simulink library "GenericTarget"  (R2025b)
settings: Solver=VariableStepAuto  StartTime=0.0  StopTime=10.0  RelTol=1e-3
undefined symbols (not defined in the file or in its folder): GT_CheckUniqueParameterValue, strlength
libraries: simulink x4, $bdroot x2, etargetslib x1
(part 1 of 3)
settings Model: Creator=damerius  LastModifiedBy=damerius
settings SolverCC: AlgebraicLoopSolver=TrustRegion
settings OptimizationCC: ReuseModelBlockBuffer=off
settings DebuggingCC: UnconnectedInputMsg=warning  UnconnectedOutputMsg=warning  UnconnectedLineMsg=warning
settings ModelReferenceCC: EnableRefExpFcnMdlSchedulingChecks=on
settings RTWCC: GPUComputeCapability=3.5  DLArmComputeVersion=19.05

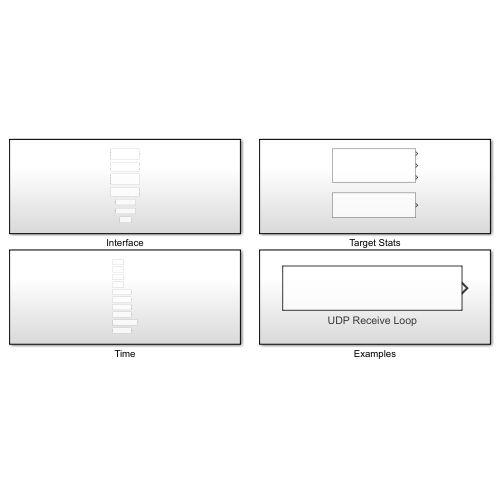
[thumbnail: Simulink's stored preview of the top-level diagram]
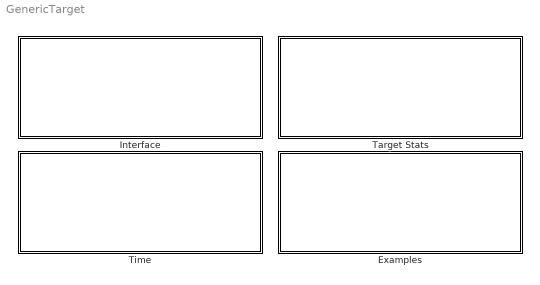
== system GenericTarget ==
  Examples : Subsystem
  Interface : Subsystem
  Target Stats : Subsystem
  Time : Subsystem

== system GenericTarget/Examples ==
  UDP Receive Loop : Subsystem  TreatAsAtomicUnit=on

== system GenericTarget/Interface ==
  Stop Execution : Subsystem  mask{SampleTime=-1}
      mask prompts: SampleTime "Sample time (-1 for inherited):"
      mask help:
      | Stop the execution of the target model. During simulation this block has no effect.<br><br>
      |
      | <b>stop</b><br>
      | True if the execution is to be stopped, false otherwise.
      mask Help: eval('GT.OpenDocumentation(''library_gt_interface_stopexecution.html'');');
      mask DialogControl DescGroupVar Prompt: Stop Execution - Generic Target
      mask Display:
      | % Get dimension of block
      | pos = get_param(gcb, 'Position');
      | width = pos(3) - pos(1);
      | height = pos(4) - pos(2);
      | 
      | % Set image to center of block
      | imgSize = 32;
      | image('GT_Icon.svg', [0.5*(width-imgSize),0.5*(height-imgSize),imgSize,imgSize]);
      | 
      | % Block title
      | text(0.5*width,0.5*(height+imgSize)+2, '{\bfStop Execution}','horizontalAlignment','center','verticalAlignment','bottom','texmode','on');
  TCP Client Receive : Subsystem  mask{showDetails=off, manageConnection=on, localPort=0, deviceName='', rxBufferSize=2048, socketPriority=6, SampleTime=-1}
      mask prompts: showDetails "Show details output port"; manageConnection "Manage connection to server"; localPort "Local port (<= 0 for dynamic port):"; deviceName "Bind to device ('' for default device):"; rxBufferSize "Receive buffer size:"; socketPriority "Socket priority (0 (lowest) ... 6 (highest), default is 6):"; SampleTime "Sample time (-1 for inherited):"
      mask help:
      | Receive data from a connected TCP server. The server address is set via the server input of a TCP Client Send or TCP Client Receive block if the <b>manageConnection</b> checkbox is enabled. For each local TCP port, a separate thread is started, that manages socket creation and connection handling to the server.<br><br>
      |
      | <b>serverAddress</b><br>A 4-dimensional vector indicating the IPv4 address of the server. A zero-value address, e.g. 0.0.0.0, disconnects the client from the server.<br><br>
      |
      | <b>serverPort</b><br>The server port. A value of 0 disconnects the client from the server.<br><br>
      |
      | <b>bytes</b><br>N-dimensional vector containing the data that has been fetched from the network buffer, where N indicates the receive buffer size.<br><br>
      |
      | <b>length</b><br>The actual number of bytes that have been received or zero in case of errors.<br><br>
      |
      | <b>details.result</b><br>Result of the socket recv function call: The number of bytes that have been received, zero if connection has been closed or a negative value in case of errors.<br><br>
      |
      | <b>details.lastErrorCode</b><br>The last socket error code from sending a message. 0 means no error. The actual meaning of non-zero values depend on the operating system.<br><br>
      |
      | <b>details.isConnected</b><br>The latest connection state to the server.
      mask init:
      | % optional details output port
      |     outPortDetails = find_system(gcb, 'LookUnderMasks','on','FollowLinks','on','Name','details');
      |     termPortDetails = find_system(gcb, 'LookUnderMasks','on','FollowLinks','on','Name','Terminator');
      |     hOut = get_param([gcb,'/BusCreator'],'PortHandles');
      |     if(showDetails)
      |         if(~isempty(termPortDetails))
      |             hIn = get_param([gcb,'/Terminator'],'PortHandles');
      |             delete_line(gcb,hOut.Outport(1),hIn.Inport(1));
      |             delete_block(termPortDetails);
      |         end
      |         if(isempty(outPortDetails))
      |             add_block('built-in/Outport',[gcb,'/details']);
      |             hIn = get_param([gcb,'/details'],'PortHandles');
      |             add_line(gcb,hOut.Outport(1),hIn.Inport(1));
      |             set_param([gcb,'/details'],'Port','3');
      |             set_param([gcb,'/details'],'Position',[25 33 55 47]);
      |         end
      |     else
      |         if(~isempty(outPortDetails))
      |             hIn = get_param([gcb,'/details'],'PortHandles');
      |             delete_line(gcb,hOut.Outport(1),hIn.Inport(1));
      |             delete_block(outPortDetails);
      |         end
      |         if(isempty(termPortDetails))
      |             add_block('built-in/Terminator',[gcb,'/Terminator']);
      |             hIn = get_param([gcb,'/Terminator'],'PortHandles');
      |             add_line(gcb,hOut.Outport(1),hIn.Inport(1));
      |             set_param([gcb,'/Terminator'],'Position',[30 30 50 50]);
      |         end
      |     end
      mask Help: eval('GT.OpenDocumentation(''library_gt_interface_tcpclientreceive.html'');');
      mask DialogControl DescGroupVar Prompt: TCP Client Receive - Generic Target
      mask DialogControl Container3 Prompt: Optional output
      mask DialogControl Container2 Prompt: Connection Management
      mask DialogControl Control2 Prompt: <i>If this checkbox is disabled, then the serverAddress and serverPort inputs are ignored.</i>
      mask DialogControl Container5 Prompt: Socket
      mask DialogControl Container6 Prompt: Advanced
      mask Display:
      | % Get dimension of block
      | pos = get_param(gcb, 'Position');
      | width = pos(3) - pos(1);
      | height = pos(4) - pos(2);
      | 
      | % Set image to center of block
      | imgSize = 32;
      | image('GT_Icon.svg', [0.5*(width-imgSize),0.5*(height-imgSize),imgSize,imgSize]);
      | 
      | % Block title
      | text(0.5*width,0.5*(height+imgSize)+2, '{\bfTCP Client Receive}','horizontalAlignment','center','verticalAlignment','bottom','texmode','on');
      | 
      | % Show socket port
      | maskStr = get_param(gcb,'localPort');
      | strText = ['Port: ' maskStr];
      | text(0.5*width,0.5*(height-imgSize)-2,strText, 'horizontalAlignment','center','verticalAlignment','top');
  TCP Client Send : Subsystem  mask{showDetails=off, manageConnection=on, localPort=0, deviceName='', socketPriority=6, SampleTime=-1}
      mask prompts: showDetails "Show details output port"; manageConnection "Manage connection to server"; localPort "Local port (<= 0 for dynamic port):"; deviceName "Bind to device ('' for default device):"; socketPriority "Socket priority (0 (lowest) ... 6 (highest), default is 6):"; SampleTime "Sample time (-1 for inherited):"
      mask help:
      | Send data to a connected TCP server. The server address is set via the server input of a TCP Client Send or TCP Client Receive block if the <b>manageConnection</b> checkbox is enabled. For each local TCP port, a separate thread is started, that manages socket creation and connection handling to the server.<br><br>
      |
      | <b>serverAddress</b><br>A 4-dimensional vector indicating the IPv4 address of the server. A zero-value address, e.g. 0.0.0.0, disconnects the client from the server.<br><br>
      |
      | <b>serverPort</b><br>The server port. A value of 0 disconnects the client from the server.<br><br>
      |
      | <b>bytes</b><br>A vector containing the data that should be sent.<br><br>
      |
      | <b>length</b><br>The number of bytes that should be sent.<br><br>
      |
      | <b>numBytesSent</b><br>The number of bytes that have been sent or zero in case of errors.<br><br>
      |
      | <b>details.result</b><br>Result of the socket send function call: The number of bytes that have been sent or a negative value in case of errors.<br><br>
      |
      | <b>details.lastErrorCode</b><br>The last socket error code from sending a message. 0 means no error. The actual meaning of non-zero values depend on the operating system.<br><br>
      |
      | <b>details.isConnected</b><br>The latest connection state to the server.
      mask init:
      | outPortDetails = find_system(gcb, 'LookUnderMasks','on','FollowLinks','on','Name','details');
      |     termPortDetails = find_system(gcb, 'LookUnderMasks','on','FollowLinks','on','Name','Terminator');
      |     hOut = get_param([gcb,'/BusCreator'],'PortHandles');
      |     if(showDetails)
      |         if(~isempty(termPortDetails))
      |             hIn = get_param([gcb,'/Terminator'],'PortHandles');
      |             delete_line(gcb,hOut.Outport(1),hIn.Inport(1));
      |             delete_block(termPortDetails);
      |         end
      |         if(isempty(outPortDetails))
      |             add_block('built-in/Outport',[gcb,'/details']);
      |             hIn = get_param([gcb,'/details'],'PortHandles');
      |             add_line(gcb,hOut.Outport(1),hIn.Inport(1));
      |             set_param([gcb,'/details'],'Port','2');
      |             set_param([gcb,'/details'],'Position',[10 33 40 47]);
      |         end
      |     else
      |         if(~isempty(outPortDetails))
      |             hIn = get_param([gcb,'/details'],'PortHandles');
      |             delete_line(gcb,hOut.Outport(1),hIn.Inport(1));
      |             delete_block(outPortDetails);
      |         end
      |         if(isempty(termPortDetails))
      |             add_block('built-in/Terminator',[gcb,'/Terminator']);
      |             hIn = get_param([gcb,'/Terminator'],'PortHandles');
      |             add_line(gcb,hOut.Outport(1),hIn.Inport(1));
      |             set_param([gcb,'/Terminator'],'Position',[15 30 35 50]);
      |         end
      |     end
      mask Help: eval('GT.OpenDocumentation(''library_gt_interface_tcpclientsend.html'');');
      mask DialogControl DescGroupVar Prompt: TCP Client Send - Generic Target
      mask DialogControl Container7 Prompt: Optional output
      mask DialogControl Container6 Prompt: Connection Management
      mask DialogControl Control2 Prompt: <i>If this checkbox is disabled, then the serverAddress and serverPort inputs are ignored.</i>
      mask DialogControl Container4 Prompt: Socket
      mask DialogControl Container5 Prompt: Advanced
      mask Display:
      | % Get dimension of block
      | pos = get_param(gcb, 'Position');
      | width = pos(3) - pos(1);
      | height = pos(4) - pos(2);
      | 
      | % Set image to center of block
      | imgSize = 32;
      | image('GT_Icon.svg', [0.5*(width-imgSize),0.5*(height-imgSize),imgSize,imgSize]);
      | 
      | % Block title
      | text(0.5*width,0.5*(height+imgSize)+2, '{\bfTCP Client Send}','horizontalAlignment','center','verticalAlignment','bottom','texmode','on');
      | 
      | % Show socket port
      | maskStr = get_param(gcb,'localPort');
      | strText = ['Port: ' maskStr];
      | text(0.5*width,0.5*(height-imgSize)-2,strText, 'horizontalAlignment','center','verticalAlignment','top');
  UDP Receive : Subsystem  mask{showDetails=off, localPort=0, deviceName='', rxBufferSize=2048, multicastGroupSource=internal, multicastGroup=[0,0,0,0], multicastTTL=1, multicastInterfaceAddress=[0,0,0,0], multicastAll=on, multicastLoop=on, socketPriority=6, allowBroadcast=off, allowZeroLengthMessage=off, fetchAll=on, SampleTime=-1}
      mask prompts: showDetails "Show details output port"; localPort "Local port (<= 0 for dynamic port):"; deviceName "Bind to device ('' for default device):"; rxBufferSize "Receive buffer size:"; multicastGroupSource "Multicast group source:"; multicastGroup "Multicast groups to join (N-by-4 matrix):"; multicastTTL "Time-to-live value for outgoing multicast traffic (default is 1):"; multicastInterfaceAddress "Multicast interface address ([0,0,0,0] for INADDR_ANY):"; multicastAll "IP_MULTICAST_ALL"; multicastLoop "IP_MULTICAST_LOOP"; socketPriority "Socket priority (0 (lowest) ... 6 (highest), default is 6):"; allowBroadcast "Allow sending broadcast message"; allowZeroLengthMessage "Allow sending zero-length message"; fetchAll "Fetch all messages from the network buffer"; SampleTime "Sample time (-1 for inherited):"
      mask help:
      | Receive a UDP message at the specified port. By default all messages from the network buffer of the operating system are fetched and only the latest message is returned. However, this option can be disabled in the advanced tab.<br><br>
      |
      | <b>bytes</b><br>N-dimensional vector containing the latest message that has been fetched from the network buffer, where N indicates the receive buffer size.<br><br>
      |
      | <b>length</b><br>The actual length of the corresponding message or zero in case of errors.<br><br>
      |
      | <b>details.sourceAddress</b><br>A 4-dimensional vector denoting the IPv4 source address of the received message.<br><br>
      |
      | <b>details.sourcePort</b><br>The source port of the received message.<br><br>
      |
      | <b>details.result</b><br>Result of the socket recvfrom function call: The number of bytes that have been received or a negative value in case of errors.<br><br>
      |
      | <b>details.lastErrorCode</b><br>The last socket error code from receiving a message. 0 means no error. The actual meaning of non-zero values depend on the operating system.<br><br>
      |
      | <b>groupsToJoin</b><br>Optional input that is enabled if the multicast group source is set to external in the multicast tab. The signal must be an N-by-4 matrix that represent N multicast group addresses to be joined. Addresses not being inside the valid multicast group address range are ignored.
      mask init:
      | % optional details output port
      |     outPortDetails = find_system(gcb, 'LookUnderMasks','on','FollowLinks','on','Name','details');
      |     termPortDetails = find_system(gcb, 'LookUnderMasks','on','FollowLinks','on','Name','Terminator');
      |     hOut = get_param([gcb,'/BusCreator'],'PortHandles');
      |     if(showDetails)
      |         if(~isempty(termPortDetails))
      |             hIn = get_param([gcb,'/Terminator'],'PortHandles');
      |             delete_line(gcb,hOut.Outport(1),hIn.Inport(1));
      |             delete_block(termPortDetails);
      |         end
      |         if(isempty(outPortDetails))
      |             add_block('built-in/Outport',[gcb,'/details']);
      |             hIn = get_param([gcb,'/details'],'PortHandles');
      |             add_line(gcb,hOut.Outport(1),hIn.Inport(1));
      |             set_param([gcb,'/details'],'Port','3');
      |             set_param([gcb,'/details'],'Position',[25 33 55 47]);
      |         end
      |     else
      |         if(~isempty(outPortDetails))
      |             hIn = get_param([gcb,'/details'],'PortHandles');
      |             delete_line(gcb,hOut.Outport(1),hIn.Inport(1));
      |             delete_block(outPortDetails);
      |         end
      |         if(isempty(termPortDetails))
      |             add_block('built-in/Terminator',[gcb,'/Terminator']);
      |             hIn = get_param([gcb,'/Terminator'],'PortHandles');
      |             add_line(gcb,hOut.Outport(1),hIn.Inport(1));
      |             set_param([gcb,'/Terminator'],'Position',[30 30 50 50]);
      |         end
      |     end
      | 
      |     % multicastGroups input port
      |     inPortGroups = find_system(gcb, 'LookUnderMasks','on','FollowLinks','on','Name','groupsToJoin');
      |     constantGroups = find_system(gcb, 'LookUnderMasks','on','FollowLinks','on','Name','constantGroupsToJoin');
      |     popupValue = get_param(gcb,'multicastGroupSource');
      |     hIn = get_param([gcb,'/Transpose'],'PortHandles');
      |     if(strcmp(popupValue,'internal'))
      |         if(~isempty(inPortGroups))
      |             hOut = get_param([gcb,'/groupsToJoin'],'PortHandles');
      |             delete_line(gcb,hOut.Outport(1),hIn.Inport(1));
      |             delete_block(inPortGroups);
      |         end
      |         if(isempty(constantGroups))
      |             add_block('built-in/Constant',[gcb,'/constantGroupsToJoin']);
      |             hOut = get_param([gcb,'/constantGroupsToJoin'],'PortHandles');
      |             add_line(gcb,hOut.Outport(1),hIn.Inport(1));
      |             set_param([gcb,'/constantGroupsToJoin'],'Value','multicastGroup');
      |             set_param([gcb,'/constantGroupsToJoin'],'Position',[-1290 -5 -1120 15]);
      |         end
      |     else
      |         if(~isempty(constantGroups))
      |             hOut = get_param([gcb,'/constantGroupsToJoin'],'PortHandles');
      |             delete_line(gcb,hOut.Outport(1),hIn.Inport(1));
      |             delete_block(constantGroups);
      |         end
      |         if(isempty(inPortGroups))
      |             add_block('built-in/Inport',[gcb,'/groupsToJoin']);
      |             hOut = get_param([gcb,'/groupsToJoin'],'PortHandles');
      |             add_line(gcb,hOut.Outport(1),hIn.Inport(1));
      |             set_param([gcb,'/groupsToJoin'],'Port','1');
      |             set_param([gcb,'/groupsToJoin'],'Position',[-1150 -2 -1120 12]);
      |         end
      |     end
      mask Help: eval('GT.OpenDocumentation(''library_gt_interface_udpreceive.html'');');
      mask Callback multicastGroupSource:
      | popupValue = get_param(gcb,'multicastGroupSource');
      |     if(strcmp(popupValue, 'internal'))
      |         set_param(gcb,'MaskEnables',{'on','on','on','on','on','on','on','on','on','on','on','on','on','on','on'});
      |     else
      |         set_param(gcb,'MaskEnables',{'on','on','on','on','on','off','on','on','on','on','on','on','on','on','on'});
      |     end
      mask DialogControl DescGroupVar Prompt: UDP Receive - Generic Target
      mask DialogControl ParameterGroupVar Prompt: Optional output
      mask DialogControl Container4 Prompt: Socket
      mask DialogControl Container5 Prompt: Multicast
      mask DialogControl Container7 Prompt: Socket options
      mask DialogControl Container6 Prompt: Advanced
      mask Display:
      | % Get dimension of block
      | pos = get_param(gcb, 'Position');
      | width = pos(3) - pos(1);
      | height = pos(4) - pos(2);
      | 
      | % Set image to center of block
      | imgSize = 32;
      | image('GT_Icon.svg', [0.5*(width-imgSize),0.5*(height-imgSize),imgSize,imgSize]);
      | 
      | % Block title
      | text(0.5*width,0.5*(height+imgSize)+2, '{\bfUDP Receive}','horizontalAlignment','center','verticalAlignment','bottom','texmode','on');
      | 
      | % Show socket port
      | maskStr = get_param(gcb,'localPort');
      | strText = ['Port: ' maskStr];
      | text(0.5*width,0.5*(height-imgSize)-2,strText, 'horizontalAlignment','center','verticalAlignment','top');
  UDP Send : Subsystem  mask{showDetails=off, localPort=0, deviceName='', multicastTTL=1, multicastInterfaceAddress=[0,0,0,0], multicastAll=on, multicastLoop=on, socketPriority=6, allowBroadcast=off, allowZeroLengthMessage=off, SampleTime=-1}
      mask prompts: showDetails "Show details output port"; localPort "Local port (<= 0 for dynamic port):"; deviceName "Bind to device ('' for default device):"; multicastTTL "Time-to-live value for outgoing multicast traffic (default is 1):"; multicastInterfaceAddress "Multicast interface address ([0,0,0,0] for INADDR_ANY):"; multicastAll "IP_MULTICAST_ALL"; multicastLoop "IP_MULTICAST_LOOP"; socketPriority "Socket priority (0 (lowest) ... 6 (highest), default is 6):"; allowBroadcast "Allow sending broadcast message"; allowZeroLengthMessage "Allow sending zero-length message"; SampleTime "Sample time (-1 for inherited):"
      mask help:
      | Send a UDP message to a destination address that is specified via the destination input. By default a message of zero-length is not sent. However, this option can be enabled in the advanced tab.<br><br>
      |
      | <b>destinationAddress</b><br>A 4-dimensional vector indicating the destination IPv4 address.<br><br>
      |
      | <b>destinationPort</b><br>The destination port.<br><br>
      |
      | <b>bytes</b><br>A vector containing the message that should be sent.<br><br>
      |
      | <b>length</b><br>The number of bytes that should be sent. The length must not be greater than 65507.<br><br>
      |
      | <b>details.result</b><br>Result of the socket sendto function call: The number of bytes that have been sent or a negative value in case of errors.<br><br>
      |
      | <b>details.lastErrorCode</b><br>The last socket error code from sending a message. 0 means no error. The actual meaning of non-zero values depend on the operating system.
      mask init:
      | outPortDetails = find_system(gcb, 'LookUnderMasks','on','FollowLinks','on','Name','details');
      |     termPortDetails = find_system(gcb, 'LookUnderMasks','on','FollowLinks','on','Name','Terminator');
      |     hOut = get_param([gcb,'/BusCreator'],'PortHandles');
      |     if(showDetails)
      |         if(~isempty(termPortDetails))
      |             hIn = get_param([gcb,'/Terminator'],'PortHandles');
      |             delete_line(gcb,hOut.Outport(1),hIn.Inport(1));
      |             delete_block(termPortDetails);
      |         end
      |         if(isempty(outPortDetails))
      |             add_block('built-in/Outport',[gcb,'/details']);
      |             hIn = get_param([gcb,'/details'],'PortHandles');
      |             add_line(gcb,hOut.Outport(1),hIn.Inport(1));
      |             set_param([gcb,'/details'],'Port','1');
      |             set_param([gcb,'/details'],'Position',[10 33 40 47]);
      |         end
      |     else
      |         if(~isempty(outPortDetails))
      |             hIn = get_param([gcb,'/details'],'PortHandles');
      |             delete_line(gcb,hOut.Outport(1),hIn.Inport(1));
      |             delete_block(outPortDetails);
      |         end
      |         if(isempty(termPortDetails))
      |             add_block('built-in/Terminator',[gcb,'/Terminator']);
      |             hIn = get_param([gcb,'/Terminator'],'PortHandles');
      |             add_line(gcb,hOut.Outport(1),hIn.Inport(1));
      |             set_param([gcb,'/Terminator'],'Position',[15 30 35 50]);
      |         end
      |     end
      mask Help: eval('GT.OpenDocumentation(''library_gt_interface_udpsend.html'');');
      mask DialogControl DescGroupVar Prompt: UDP Send - Generic Target
      mask DialogControl ParameterGroupVar Prompt: Optional output
      mask DialogControl Container4 Prompt: Socket
      mask DialogControl Container6 Prompt: Multicast
      mask DialogControl Container7 Prompt: Socket options
      mask DialogControl Container5 Prompt: Advanced
      mask Display:
      | % Get dimension of block
      | pos = get_param(gcb, 'Position');
      | width = pos(3) - pos(1);
      | height = pos(4) - pos(2);
      | 
      | % Set image to center of block
      | imgSize = 32;
      | image('GT_Icon.svg', [0.5*(width-imgSize),0.5*(height-imgSize),imgSize,imgSize]);
      | 
      | % Block title
      | text(0.5*width,0.5*(height+imgSize)+2, '{\bfUDP Send}','horizontalAlignment','center','verticalAlignment','bottom','texmode','on');
      | 
      | % Show socket port
      | maskStr = get_param(gcb,'localPort');
      | strText = ['Port: ' maskStr];
      | text(0.5*width,0.5*(height-imgSize)-2,strText, 'horizontalAlignment','center','verticalAlignment','top');
  Write Bus To File : Subsystem  InitFcn=GT_CheckUniqueParameterValue(gcs,gcb,'strID');  mask{strID='myData', numSamplesPerFile=0, threadPriority=30, writeFilesDuringSimulation=off, SampleTime=-1, numBytesPerSample=8, strSignalNames='a', strlenSignalNames=1, strDimensions='[1]', strlenDimensions=3, strDataTypes='double', strlenDataTypes=6}
      mask prompts: strID "Unique ID:"; numSamplesPerFile "Number of samples per file (0 for infinite samples):"; threadPriority "Thread priority in range [1 (lowest), 99 (highest)]:"; writeFilesDuringSimulation "write files during simulation"; SampleTime "Sample time (-1 for inherited):"
      mask help: Write a complete bus signal to a file. Internally a digital clock is used as timestamp. The number of samples to be written into a single file can be specified. A sample indicates a data vector of all signals in the bus and the timestamp for one sample time point.
      mask init:
      | GT_WriteBusToFileInitFcn(gcb);
      mask Help: eval('GT.OpenDocumentation(''library_gt_interface_writebustofile.html'');');
      mask DialogControl DescGroupVar Prompt: Write Bus To File - Generic Target
      mask DialogControl Container3 Prompt: Bus input
      mask DialogControl Control3 Prompt: Connect a bus signal to the input port and click the "Update" button. Make sure that the model can be compiled successfully.
      mask DialogControl buttonUpdate Prompt: Update
      mask DialogControl buttonUpdate Callback: GT_UpdateWriteBusToFile(gcb);
      mask DialogControl Control4 Prompt: <p style="color: #f00;"><b>NOTE:</b> You must not use multiple Write To File blocks with the <u>same</u> ID!</p>
      mask DialogControl Control5 Prompt: If this option is enabled, a data folder is created to the current working directory whenever the initialization callback is triggered.
      mask DialogControl Container5 Prompt: Hidden Parameters
      mask Display:
      | % Get dimension of block
      | pos = get_param(gcb, 'Position');
      | width = pos(3) - pos(1);
      | height = pos(4) - pos(2);
      | 
      | % Set image to center of block
      | imgSize = 32;
      | image('GT_Icon.svg', [0.5*(width-imgSize),0.5*(height-imgSize),imgSize,imgSize]);
      | 
      | % Block title
      | text(0.5*width,0.5*(height+imgSize)+2, '{\bfWrite Bus To File}','horizontalAlignment','center','verticalAlignment','bottom','texmode','on');
      | 
      | % Show ID
      | maskStr = get_param(gcb,'strID');
      | text(4,2,['ID: ',maskStr],'horizontalAlignment','left','verticalAlignment','bottom');
  Write Scalar Doubles To File : Subsystem  InitFcn=GT_CheckUniqueParameterValue(gcs,gcb,'strID');  mask{strID='myData', numSamplesPerFile=0, threadPriority=30, writeFilesDuringSimulation=off, numSignals=2, signalNames=signal1,signal2, numCharacters=15, SampleTime=-1}
      mask prompts: strID "Unique ID:"; numSamplesPerFile "Number of samples per file (0 for infinite samples):"; threadPriority "Thread priority in range [1 (lowest), 99 (highest)]:"; writeFilesDuringSimulation "write files during simulation"; SampleTime "Sample time (-1 for inherited):"
      mask help:
      | Write a bus signal of scalar doubles to a file. Internally, a digital clock is used as timestamp. The number of samples to be written into one file can be specified. A sample indicates a vector of values including the time and all signals in the bus.<br>
      | <p style="color: #f00;"><b>NOTE:</b> The input <u>must</u> be connected to a bus that only contains scalar values of type double! Otherwise, the mask initialization function is going to fail.</p>
      | If structural changes have been made to the input bus, it may be necessary to update the model twice.
      mask init:
      | GT_WriteScalarDoublesToFileInitFcn(gcb);
      mask Help: eval('GT.OpenDocumentation(''library_gt_interface_writescalardoublestofile.html'');');
      mask DialogControl DescGroupVar Prompt: Write Scalar Doubles To File - Generic Target
      mask DialogControl Control2 Prompt: <p style="color: #f00;"><b>NOTE:</b> You must not use multiple Write To File blocks with the <u>same</u> ID!</p>
      mask DialogControl Control3 Prompt: If this option is enabled, a data folder is created to the current working directory whenever the initialization callback is triggered.
      mask Display:
      | % Get dimension of block
      | pos = get_param(gcb, 'Position');
      | width = pos(3) - pos(1);
      | height = pos(4) - pos(2);
      | 
      | % Set image to center of block
      | imgSize = 32;
      | image('GT_Icon.svg', [0.5*(width-imgSize),0.5*(height-imgSize),imgSize,imgSize]);
      | 
      | % Block title
      | text(0.5*width,0.5*(height+imgSize)+2, '{\bfWrite Scalar Doubes To File}','horizontalAlignment','center','verticalAlignment','bottom','texmode','on');
      | 
      | % Show ID
      | maskStr = get_param(gcb,'strID');
      | text(4,2,['ID: ',maskStr],'horizontalAlignment','left','verticalAlignment','bottom');

== system GenericTarget/Target Stats ==
  Application Arguments : Subsystem  mask{maxNumCharsPerArgument=32, maxNumArguments=8, SampleTime=-1}
      mask prompts: maxNumCharsPerArgument "Maximum number of characters per argument:"; maxNumArguments "Maximum number of arguments:"; SampleTime "Sample time (-1 for inherited):"
      mask help:
      | Get all arguments that have been passed to the application. The first argument is the executable name. The maximum number of characters as well as the maximum number of arguments that can be stored in the output are configured via the block mask. During simulation this block has no effect.<br><br>
      | <b>args</b><br>
      | N-by-M matrix of type uint8, where N and M indicate the maximum number of characters per argument and the maximum number of arguments, respectively.
      | <br><br>
      | <b>numCharacters</b><br>
      | M-dimensional vector of type uint32, where each element indicates the actual number of characters that represent the argument in the M-th column of the <i>args</i> output matrix.
      | <br><br>
      | <b>numArguments</b><br>
      | Scalar value of type uint32 indicating the actual number of arguments present in the <i>args</i> output matrix.
      mask Help: eval('GT.OpenDocumentation(''library_gt_targetstats_applicationarguments.html'');');
      mask DialogControl DescGroupVar Prompt: Application Arguments
      mask Display:
      | % Get dimension of block
      | pos = get_param(gcb, 'Position');
      | width = pos(3) - pos(1);
      | height = pos(4) - pos(2);
      | 
      | % Set image to center of block
      | imgSize = 32;
      | image('GT_Icon.svg', [0.5*(width-imgSize),0.5*(height-imgSize),imgSize,imgSize]);
      | 
      | % Block title
      | text(width/2, height, '{\bfApplication Arguments}','horizontalAlignment','center','verticalAlignment','top','texmode','on');
  Read Thermal Zones : Subsystem  mask{maxNumThermalZones=8, SampleTime=-1}
      mask prompts: maxNumThermalZones "Maximum number of thermal zones:"; SampleTime "Sample time (-1 for inherited):"
      mask help: Read all temperature values from "/sys/class/thermal/thermal_zone[i]/temp" with [i] being the index of the thermal zone. The maximum number of thermal zones to read from is specified via the mask parameter. The output dimension is equal to that number. If a thermal zone does not exist, NaN is returned for the corresponding index. This block has no effect on a non-linux OS.
      mask Help: eval('GT.OpenDocumentation(''library_gt_targetstats_readthermalzones.html'');');
      mask DialogControl DescGroupVar Prompt: Read Thermal Zones - Generic Target
      mask Display:
      | % Get dimension of block
      | pos = get_param(gcb, 'Position');
      | width = pos(3) - pos(1);
      | height = pos(4) - pos(2);
      | 
      | % Set image to center of block
      | imgSize = 32;
      | image('GT_Icon.svg', [0.5*(width-imgSize),0.5*(height-imgSize),imgSize,imgSize]);
      | 
      | % Block title
      | text(width/2, height, '{\bfRead Thermal Zones}','horizontalAlignment','center','verticalAlignment','top','texmode','on');

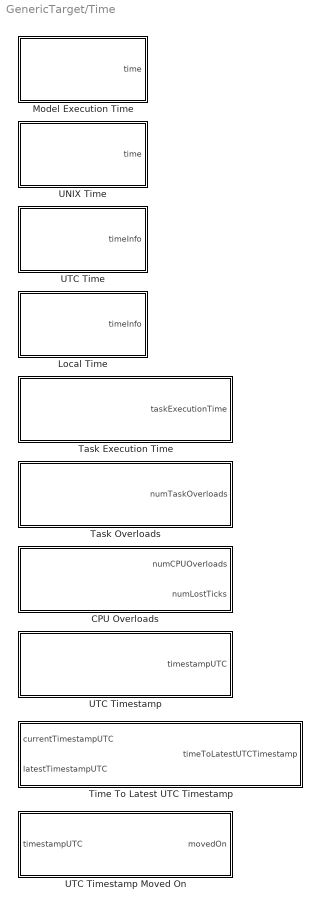
== system GenericTarget/Time ==
  CPU Overloads : Subsystem  mask{SampleTime=-1}
      mask prompts: SampleTime "Sample time (-1 for inherited):"
      mask help:
      | Get the total number of CPU overloads and lost ticks since the model has been started. During simulation this block has no effect.<br><br>
      | <b>numCPUOverloads</b><br>
      | The total number of CPU overloads that have been occurred. This value is incremented by one, if the timer interrupt event for the base rate scheduler (with the base sampletime of the model) has been lost.
      | <br><br>
      | <b>numLostTicks</b><br>
      | The total number of lost ticks from the timer. This value is incremented by the number of lost timer interrupt events.
      mask Help: eval('GT.OpenDocumentation(''library_gt_time_cpuoverloads.html'');');
      mask DialogControl DescGroupVar Prompt: CPU Overloads - Generic Target
      mask Display:
      | % Get dimension of block
      | pos = get_param(gcb, 'Position');
      | width = pos(3) - pos(1);
      | height = pos(4) - pos(2);
      | 
      | % Set image to center of block
      | imgSize = 32;
      | image('GT_Icon.svg', [0.5*(width-imgSize),0.5*(height-imgSize),imgSize,imgSize]);
      | 
      | % Block title
      | text(width/2, height, '{\bfCPU Overloads}','horizontalAlignment','center','verticalAlignment','top','texmode','on');
  Local Time : Subsystem  mask{SampleTime=-1}
      mask prompts: SampleTime "Sample time (-1 for inherited):"
      mask help:
      | Get the current local time from the system clock.<br><br>
      |
      | <b>timeInfo.nanoseconds</b><br>Nanoseconds after the second [0, 999999999].<br><br>
      |
      | <b>timeInfo.second</b><br>Seconds after the minute [0, 59] (on some systems [0,60] or [0,61] to allow leap seconds).<br><br>
      |
      | <b>timeInfo.minute</b><br>Minutes after the hour [0, 59].<br><br>
      |
      | <b>timeInfo.hour</b><br>Hours since midnight [0, 23].<br><br>
      |
      | <b>timeInfo.mday</b><br>Day of the month [1, 31].<br><br>
      |
      | <b>timeInfo.mon</b><br>Month since January [0, 11].<br><br>
      |
      | <b>timeInfo.year</b><br>Years since 1900.<br><br>
      |
      | <b>timeInfo.wday</b><br>Days since Sunday [0, 6].<br><br>
      |
      | <b>timeInfo.yday</b><br>Days since January 1 [0, 365].<br><br>
      |
      | <b>timeInfo.isdst</b><br>Daylight Saving Time flag. The value is positive if DST is in effect, zero if not and negative if no information is available.
      mask Help: eval('GT.OpenDocumentation(''library_gt_time_localtime.html'');');
      mask DialogControl DescGroupVar Prompt: Local Time - Generic Target
      mask Display:
      | % Get dimension of block
      | pos = get_param(gcb, 'Position');
      | width = pos(3) - pos(1);
      | height = pos(4) - pos(2);
      | 
      | % Set image to center of block
      | imgSize = 32;
      | image('GT_Icon.svg', [0.5*(width-imgSize),0.5*(height-imgSize),imgSize,imgSize]);
      | 
      | % Block title
      | text(width/2, height, '{\bfLocal Time}','horizontalAlignment','center','verticalAlignment','top','texmode','on');
  Model Execution Time : Subsystem  mask{SampleTime=-1}
      mask prompts: SampleTime "Sample time (-1 for inherited):"
      mask help:
      | Get the current model execution time. A steady clock is used to measure the execution time, that is, the elapsed time to the starting timepoint of the scheduler. During simulation, the output represents the measured time to some initial timepoint at the start of the simulation.<br><br>
      |
      | <b>time</b><br>The model execution time in seconds.
      mask Help: eval('GT.OpenDocumentation(''library_gt_time_modelexecutiontime.html'');');
      mask DialogControl DescGroupVar Prompt: Model Execution Time - Generic Target
      mask Display:
      | % Get dimension of block
      | pos = get_param(gcb, 'Position');
      | width = pos(3) - pos(1);
      | height = pos(4) - pos(2);
      | 
      | % Set image to center of block
      | imgSize = 32;
      | image('GT_Icon.svg', [0.5*(width-imgSize),0.5*(height-imgSize),imgSize,imgSize]);
      | 
      | % Block title
      | text(width/2, height, '{\bfModel Execution Time}','horizontalAlignment','center','verticalAlignment','top','texmode','on');
  Task Execution Time : Subsystem  mask{strTaskName='D1', SampleTime=-1}
      mask prompts: strTaskName "Task name, e.g. 'D1':"; SampleTime "Sample time (-1 for inherited):"
      mask help: Get the current task execution time in seconds for the task with the specified name. If this task does not exist, zero is returned. During simulation this block has no effect.
      mask Help: eval('GT.OpenDocumentation(''library_gt_time_taskexecutiontime.html'');');
      mask DialogControl DescGroupVar Prompt: Task Execution Time - Generic Target
      mask Display:
      | % Get dimension of block
      | pos = get_param(gcb, 'Position');
      | width = pos(3) - pos(1);
      | height = pos(4) - pos(2);
      | 
      | % Set image to center of block
      | imgSize = 32;
      | image('GT_Icon.svg', [0.5*(width-imgSize),0.5*(height-imgSize),imgSize,imgSize]);
      | 
      | % Block title
      | text(width/2, height, '{\bfTask Execution Time}','horizontalAlignment','center','verticalAlignment','top','texmode','on');
      | 
      | % Show task name
      | maskStr = get_param(gcb,'strTaskName');
      | text(4,2,['Task: ',maskStr],'horizontalAlignment','left','verticalAlignment','bottom');
  Task Overloads : Subsystem  mask{strTaskName='D1', SampleTime=-1}
      mask prompts: strTaskName "Task name, e.g. 'D1':"; SampleTime "Sample time (-1 for inherited):"
      mask help: Get the total number of task overloads for the task with the specified name. If this task does not exist, zero is returned. During simulation this block has no effect.
      mask Help: eval('GT.OpenDocumentation(''library_gt_time_taskoverloads.html'');');
      mask DialogControl DescGroupVar Prompt: Task Overloads - Generic Target
      mask Display:
      | % Get dimension of block
      | pos = get_param(gcb, 'Position');
      | width = pos(3) - pos(1);
      | height = pos(4) - pos(2);
      | 
      | % Set image to center of block
      | imgSize = 32;
      | image('GT_Icon.svg', [0.5*(width-imgSize),0.5*(height-imgSize),imgSize,imgSize]);
      | 
      | % Block title
      | text(width/2, height, '{\bfTask Overloads}','horizontalAlignment','center','verticalAlignment','top','texmode','on');
      | 
      | % Show task name
      | maskStr = get_param(gcb,'strTaskName');
      | text(4,2,['Task: ',maskStr],'horizontalAlignment','left','verticalAlignment','bottom');
  Time To Latest UTC Timestamp : Subsystem
      mask help:
      | This block calculates the time difference (seconds) to the latest UTC timestamp taking into account the wrap range of the UTC timestamp.<br><br>
      | The basic behaviour is as follows:<br>
      | <b>output</b> = <b>current</b> - <b>latest</b>
      mask Help: eval('GT.OpenDocumentation(''library_gt_time_timetolatestutctimestamp.html'');');
      mask DialogControl DescGroupVar Prompt: Time To Latest UTC Timestamp - Generic Target
      mask Display:
      | % Get dimension of block
      | pos = get_param(gcb, 'Position');
      | width = pos(3) - pos(1);
      | height = pos(4) - pos(2);
      | 
      | % Set image to center of block
      | imgSize = 32;
      | image('GT_Icon.svg', [0.5*(width-imgSize),0.5*(height-imgSize),imgSize,imgSize]);
      | 
      | % Block title
      | text(width/2, height, '{\bfTime To Latest UTC Timestamp}','horizontalAlignment','center','verticalAlignment','top','texmode','on');
  UNIX Time : Subsystem  mask{SampleTime=-1}
      mask prompts: SampleTime "Sample time (-1 for inherited):"
      mask help:
      | Get the current UNIX time from the system clock.<br><br>
      |
      | <b>time</b><br>The UNIX time in seconds. The resolution is one millisecond.
      mask Help: eval('GT.OpenDocumentation(''library_gt_time_unixtime.html'');');
      mask DialogControl DescGroupVar Prompt: UNIX Time - Generic Target
      mask Display:
      | % Get dimension of block
      | pos = get_param(gcb, 'Position');
      | width = pos(3) - pos(1);
      | height = pos(4) - pos(2);
      | 
      | % Set image to center of block
      | imgSize = 32;
      | image('GT_Icon.svg', [0.5*(width-imgSize),0.5*(height-imgSize),imgSize,imgSize]);
      | 
      | % Block title
      | text(width/2, height, '{\bfUNIX Time}','horizontalAlignment','center','verticalAlignment','top','texmode','on');
  UTC Time : Subsystem  mask{SampleTime=-1}
      mask prompts: SampleTime "Sample time (-1 for inherited):"
      mask help:
      | Get the current UTC time from the system clock.<br><br>
      |
      | <b>timeInfo.nanoseconds</b><br>Nanoseconds after the second [0, 999999999].<br><br>
      |
      | <b>timeInfo.second</b><br>Seconds after the minute [0, 59] (on some systems [0,60] or [0,61] to allow leap seconds).<br><br>
      |
      | <b>timeInfo.minute</b><br>Minutes after the hour [0, 59].<br><br>
      |
      | <b>timeInfo.hour</b><br>Hours since midnight [0, 23].<br><br>
      |
      | <b>timeInfo.mday</b><br>Day of the month [1, 31].<br><br>
      |
      | <b>timeInfo.mon</b><br>Month since January [0, 11].<br><br>
      |
      | <b>timeInfo.year</b><br>Years since 1900.<br><br>
      |
      | <b>timeInfo.wday</b><br>Days since Sunday [0, 6].<br><br>
      |
      | <b>timeInfo.yday</b><br>Days since January 1 [0, 365].<br><br>
      |
      | <b>timeInfo.isdst</b><br>Daylight Saving Time flag. The value is positive if DST is in effect, zero if not and negative if no information is available.
      mask Help: eval('GT.OpenDocumentation(''library_gt_time_utctime.html'');');
      mask DialogControl DescGroupVar Prompt: UTC Time - Generic Target
      mask Display:
      | % Get dimension of block
      | pos = get_param(gcb, 'Position');
      | width = pos(3) - pos(1);
      | height = pos(4) - pos(2);
      | 
      | % Set image to center of block
      | imgSize = 32;
      | image('GT_Icon.svg', [0.5*(width-imgSize),0.5*(height-imgSize),imgSize,imgSize]);
      | 
      | % Block title
      | text(width/2, height, '{\bfUTC Time}','horizontalAlignment','center','verticalAlignment','top','texmode','on');
  UTC Timestamp : Subsystem  mask{SampleTime=-1}
      mask prompts: SampleTime "Sample time (-1 for inherited):"
      mask help:
      | Get the current UTC timestamp from the system clock.<br><br>
      |
      | <b>timestampUTC</b><br>UTC second of the day in range [0,86400) (on some systems [0,86401) or [0,86402) to allow leap seconds).
      mask Help: eval('GT.OpenDocumentation(''library_gt_time_utctimestamp.html'');');
      mask DialogControl DescGroupVar Prompt: UTC Timestamp - Generic Target
      mask Display:
      | % Get dimension of block
      | pos = get_param(gcb, 'Position');
      | width = pos(3) - pos(1);
      | height = pos(4) - pos(2);
      | 
      | % Set image to center of block
      | imgSize = 32;
      | image('GT_Icon.svg', [0.5*(width-imgSize),0.5*(height-imgSize),imgSize,imgSize]);
      | 
      | % Block title
      | text(width/2, height, '{\bfUTC Timestamp}','horizontalAlignment','center','verticalAlignment','top','texmode','on');
  UTC Timestamp Moved On : Subsystem  mask{vinit=0}
      mask prompts: vinit "Initial condition:"
      mask help: If the input UTC timestamp has moved on, then TRUE is returned, otherwise FALSE is returned. The initial condition determines the initial value of the previous input.
      mask Help: eval('GT.OpenDocumentation(''library_gt_time_utctimestampmovedon.html'');');
      mask DialogControl DescGroupVar Prompt: UTC Timestamp Moved On - Generic Target
      mask DialogControl Container2 Prompt: Parameters
      mask Display:
      | % Get dimension of block
      | pos = get_param(gcb, 'Position');
      | width = pos(3) - pos(1);
      | height = pos(4) - pos(2);
      | 
      | % Set image to center of block
      | imgSize = 32;
      | image('GT_Icon.svg', [0.5*(width-imgSize),0.5*(height-imgSize),imgSize,imgSize]);
      | 
      | % Block title
      | text(width/2,height, '{\bfUTC Timestamp Moved On}','horizontalAlignment','center','verticalAlignment','top','texmode','on');

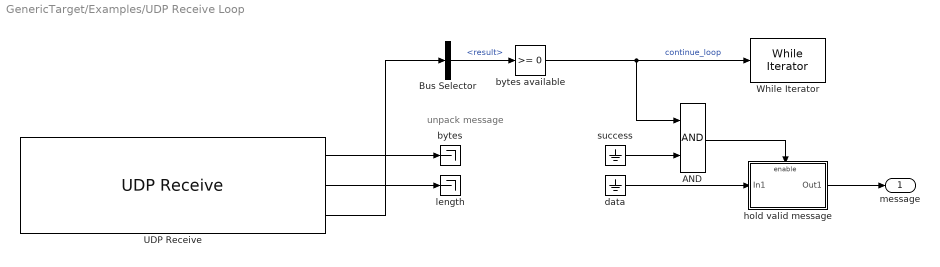
== system GenericTarget/Examples/UDP Receive Loop ==
  note: unpack message
  AND : Logic  AllPortsSameDT=off  OutDataTypeStr=boolean
  Bus Selector : BusSelector  OutputSignals=result
  UDP Receive : $bdroot/Interface/UDP Receive  showDetails=on  localPort=0  deviceName=''  rxBufferSize=2048  multicastGroupSource=internal  multicastGroup=[0,0,0,0]  multicastTTL=1  multicastInterfaceAddress=[0,0,0,0]  multicastAll=on  multicastLoop=on  socketPriority=6  allowBroadcast=off  allowZeroLengthMessage=off  fetchAll=off  SampleTime=-1
  While Iterator : WhileIterator  MaxIters=-1  WhileBlockType=do-while
  bytes : Terminator
  bytes available : simulink/Logic and Bit Operations/Compare To Zero  relop=>=  OutDataTypeStr=boolean
  data : Ground
  hold valid message : Subsystem  TreatAsAtomicUnit=on
  length : Terminator
  success : Ground
  message : Outport
  wires:
  UDP Receive/1 -> bytes/1
  UDP Receive/2 -> length/1
  UDP Receive/3 -> Bus Selector/1
  success/1 -> AND/2
  Bus Selector/1 -> bytes available/1  "<result>"
  bytes available/1 -> AND/1, While Iterator/1  "continue_loop"
  data/1 -> hold valid message/1(In1)
  hold valid message/1(Out1) -> message/1
  AND/1 -> hold valid message/Enable

== system GenericTarget/Interface/Stop Execution ==
  stop : Inport  OutDataTypeStr=boolean  PortDimensions=1
  Data Type Conversion : DataTypeConversion  OutDataTypeStr=uint8  SaturateOnIntegerOverflow=off  RndMeth=Floor
  SFunctionGTDriverStopExecution : S-Function  FunctionName=SFunctionGTDriverStopExecution  Parameters=SampleTime  SFunctionDeploymentMode=off  EnableBusSupport=off  mask(Legacy Function){SFunctionSpec=void GT_DriverStopExecutionStep(uint8 u1), SampleTime=SampleTime, ShowSpec=on}
      mask prompts: SampleTime "Sample time (-1 for inherited):"; ShowSpec "Display function specification"
      mask help:
      | This block allows you to call the legacy functions specified by the following Legacy Code Tool definition:
      | def.SFunctionName = 'SFunctionGTDriverStopExecution';
      | def.OutputFcnSpec = 'void GT_DriverStopExecutionStep(uint8 u1)';
      | def.StartFcnSpec = 'void GT_DriverStopExecutionInitialize()';
      | def.TerminateFcnSpec = 'void GT_DriverStopExecutionTerminate()';
      | def.HeaderFiles = {'GT_DriverStopExecution.hpp'};
      | def.SourceFiles = {'GT_DriverStopExecution.cpp'};
      | def.SampleTime = 'parameterized';
      | def.Options.useTlcWithAccel = false;
      | def.Options.language = 'C++';
      mask Help: <p>This block was generated automatically by the Legacy Code Tool. For detailed help on this tool, call<a href="matlab:legacy_code('help')"> legacy_code('help')</a>.</p>
      mask Callback ShowSpec:
      | if strcmp(get_param(gcbh, 'ShowSpec'), 'on')
      |   set_param(gcbh, 'MaskDisplay', sprintf('fprintf(''%s'');', get_param(gcbh, 'SFunctionSpec')));
      | else
      |   set_param(gcbh, 'MaskDisplay', sprintf('fprintf(''%s'');', get_param(gcbh, 'FunctionName')));
      | end
      mask Display: fprintf('void GT_DriverStopExecutionStep(uint8 u1)');
  wires:
  Data Type Conversion/1 -> SFunctionGTDriverStopExecution/1
  stop/1 -> Data Type Conversion/1
